simulink model "assign"  (Simulink 6.4)
settings: Solver=ode45  StartTime=0.0  StopTime=210  RelTol=1e-3
libraries: simulink x1
CloseFcn:
  | rtwprivate ssgensfun ModelCloseRequest nlgentpl
settings Model: Creator=lbusoniu  LastModifiedBy=Administrator  ExtModeAutoUpdateStatusClock=off  BufferReuse=off
settings DataIOCC: SaveOutput=off  SaveTime=off  SignalLoggingName=sigsOut
settings OptimizationCC: OptimizeBlockIOStorage=off  BufferReuse=off  ExpressionFolding=off  LocalBlockOutputs=off
settings DebuggingCC: SolverPrmCheckMsg=none  StrictBusMsg=None
settings HardwareCC: TargetUnknown=on

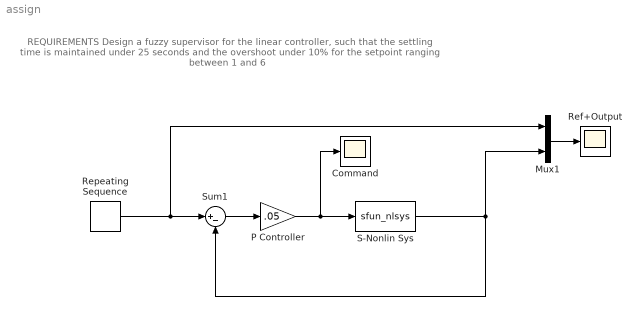
== system assign ==
  note: REQUIREMENTS
      | Design a fuzzy supervisor for the linear controller, such that
      | the settling time is maintained under 25 seconds and the overshoot under 10%
      | for the setpoint ranging between 1 and 6
  Command : Scope
      settings: TimeRange=250  YMin=-0.2  YMax=0.2  SaveName=u  DataFormat=Array
  Mux1 : Mux  Inputs=2
  P Controller : Gain  Gain=.05  SaturateOnIntegerOverflow=on
  Ref+Output : Scope
      settings: TimeRange=250  YMin=1  YMax=7  SaveName=u2  DataFormat=Array
  Repeating Sequence : simulink/Sources/Repeating Sequence  SystemSampleTime=-1  rep_seq_t=[0 30 30.5 60 60.5 90 90.5 120 120.5 150 150.5 180 180.5 211]  rep_seq_y=[4 4 1 1 3 3 2 2 5 5 3 3 6 6]
  S-Nonlin Sys : S-Function  FunctionName=sfun_nlsys
  Sum1 : Sum  Inputs=|+-  SaturateOnIntegerOverflow=on
  wires:
  Sum1/1 -> P Controller/1
  S-Nonlin Sys/1 -> Sum1/2, Mux1/2
  P Controller/1 -> S-Nonlin Sys/1, Command/1
  Mux1/1 -> Ref+Output/1
  Repeating Sequence/1 -> Sum1/1, Mux1/1
